simulink model "four_feet_simple_cdh"  (R2022b)
settings: Solver=FixedStepAuto  StartTime=0.0  StopTime=4  FixedStep=1e-4  MaxStep=1e-4  MinStep=1e-4  RelTol=1e-3  AbsTol=1e-3  EnableMultiTasking=on
undefined symbols (not defined in the file or in its folder): X, Y, Z
libraries: sm_lib x18, nesl_utility x7
settings Model: Creator=Administrator  LastModifiedBy=LiAn
settings SolverCC: AutoScaleAbsTol=off  AlgebraicLoopSolver=TrustRegion  MaxZcPerStep=1
settings DataIOCC: LimitDataPoints=on  MaxDataPoints=10000
settings OptimizationCC: LifeSpan=inf
settings DebuggingCC: UnconnectedInputMsg=warning  UnconnectedOutputMsg=warning  UnconnectedLineMsg=warning  AllowSymbolicDim=off  SFUnexpectedBacktrackingDiag=warning  SFNoUnconditionalDefaultTransitionDiag=warning  SFExecutionAtInitializationDiag=none  SFMachineParentedDataDiag=warning  ArithmeticOperatorsInVariantConditions=warning
settings ModelReferenceCC: EnableRefExpFcnMdlSchedulingChecks=on
settings SFSimCC: SimUseLocalCustomCode=off  CustomCodeUndefinedFunction=UseInterfaceOnly
settings RTWCC: RTWUseLocalCustomCode=off  DLArmComputeVersion=19.05
settings CodeAppCC: StateflowObjectComments=on
settings GRTTargetCC: TargetLangStandard=C89/C90 (ANSI)
settings ConfigComp: CovMetricSettings=dw  CovSaveCumulativeToWorkspaceVar=on  CovSaveSingleToWorkspaceVar=on  CovExternalEMLEnable=off  CovSFcnEnable=off
settings SimscapeCC: SimscapeLogType=all  SimscapeLogSimulationStatistics=on  SimscapeLogDataHistory=10000
settings DiagnosticsConfigSet: SimMechanicsRigidlyBoundBlock=warning

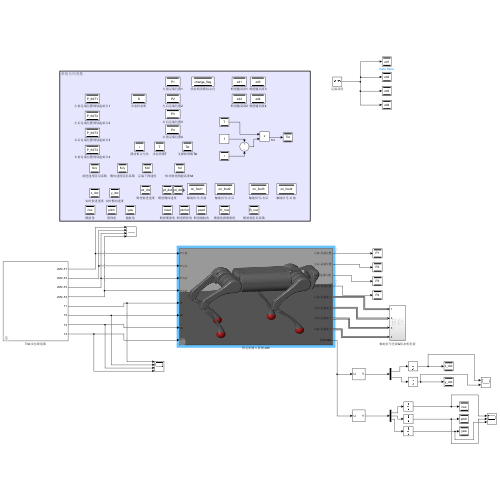
[thumbnail: Simulink's stored preview of the top-level diagram]
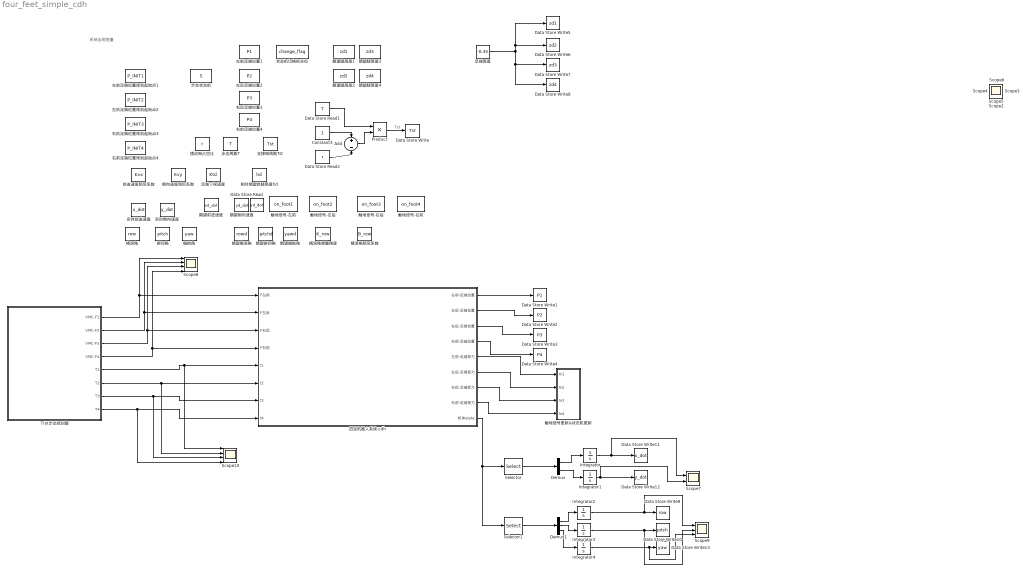
== system four_feet_simple_cdh ==
  note: 系统全局变量
  Add : Sum  Inputs=+-
  Constant3 : Constant
  Data Store Read : DataStoreRead  DataStoreName=yd_dot  IndexOptions=Index vector (dialog)  Indices=1  OutputSizes=1
  Data Store Read1 : DataStoreRead  DataStoreName=T  IndexOptions=Index vector (dialog)  Indices=1  OutputSizes=1
  Data Store Read2 : DataStoreRead  DataStoreName=r  IndexOptions=Index vector (dialog)  Indices=1  OutputSizes=1
  Data Store Write : DataStoreWrite  DataStoreName=Tst  IndexOptions=Index vector (dialog)  Indices=1  OutputSizes=1
  Data Store Write1 : DataStoreWrite  DataStoreName=P1  IndexOptions=Index vector (dialog)  Indices=1  OutputSizes=1
  Data Store Write10 : DataStoreWrite  DataStoreName=pitch  IndexOptions=Index vector (dialog)  Indices=1  OutputSizes=1
  Data Store Write11 : DataStoreWrite  DataStoreName=x_dot  IndexOptions=Index vector (dialog)  Indices=1  OutputSizes=1
  Data Store Write12 : DataStoreWrite  DataStoreName=y_dot  IndexOptions=Index vector (dialog)  Indices=1  OutputSizes=1
  Data Store Write13 : DataStoreWrite  DataStoreName=yaw  IndexOptions=Index vector (dialog)  Indices=1  OutputSizes=1
  Data Store Write2 : DataStoreWrite  DataStoreName=P2  IndexOptions=Index vector (dialog)  Indices=1  OutputSizes=1
  Data Store Write3 : DataStoreWrite  DataStoreName=P3  IndexOptions=Index vector (dialog)  Indices=1  OutputSizes=1
  Data Store Write4 : DataStoreWrite  DataStoreName=P4  IndexOptions=Index vector (dialog)  Indices=1  OutputSizes=1
  Data Store Write5 : DataStoreWrite  DataStoreName=zd1  IndexOptions=Index vector (dialog)  Indices=1  OutputSizes=1
  Data Store Write6 : DataStoreWrite  DataStoreName=zd2  IndexOptions=Index vector (dialog)  Indices=1  OutputSizes=1
  Data Store Write7 : DataStoreWrite  DataStoreName=zd3  IndexOptions=Index vector (dialog)  Indices=1  OutputSizes=1
  Data Store Write8 : DataStoreWrite  DataStoreName=zd4  IndexOptions=Index vector (dialog)  Indices=1  OutputSizes=1
  Data Store Write9 : DataStoreWrite  DataStoreName=row  IndexOptions=Index vector (dialog)  Indices=1  OutputSizes=1
  Demux : Demux  Outputs=2
  Demux1 : Demux  Outputs=3
  Integrator{,1..4} (5 alike) : Integrator
  Product : Product
  Scope10 : Scope  NumInputPorts=4
  Scope7 : Scope  NumInputPorts=2
  Scope8 : Scope  NumInputPorts=4
  Scope9 : Scope  NumInputPorts=3
  Selector : Selector  InputPortWidth=6  IndexOptions=Index vector (dialog)  Indices=[1 2]  OutputSizes=1
  Selector1 : Selector  InputPortWidth=6  IndexOptions=Index vector (dialog)  Indices=[4 5 6]  OutputSizes=1
  Trot步态规划器 : Subsystem  mask{P=2000, D=5}
      mask prompts: P "比例系数P"; D "阻尼系数D"
      mask DialogControl ParameterGroupVar Prompt: 参数
  侧向速度阻尼系数 : DataStoreMemory  DataStoreName=Kvy  WriteAfterWriteMsg=warning  InitialValue=-0.05  ShowAdditionalParam=off
  俯仰角 : DataStoreMemory  DataStoreName=pitch  WriteAfterWriteMsg=warning  ShowAdditionalParam=off
  偏航角 : DataStoreMemory  DataStoreName=yaw  WriteAfterWriteMsg=warning  ShowAdditionalParam=off
  前进速度阻尼系数 : DataStoreMemory  DataStoreName=Kvx  WriteAfterWriteMsg=warning  InitialValue=-0.3  ShowAdditionalParam=off
  右前足端位置4 : DataStoreMemory  DataStoreName=P4  WriteAfterWriteMsg=warning  InitialValue=[0 -0.085 -0.3]  ShowAdditionalParam=off
  右前足端位置规划起始点4 : DataStoreMemory  DataStoreName=P_INIT4  WriteAfterWriteMsg=warning  InitialValue=[0 -0.085 -0.3]  ShowAdditionalParam=off
  右后足端位置3 : DataStoreMemory  DataStoreName=P3  WriteAfterWriteMsg=warning  InitialValue=[0 -0.085 -0.3]  ShowAdditionalParam=off
  右后足端位置规划起始点3 : DataStoreMemory  DataStoreName=P_INIT3  WriteAfterWriteMsg=warning  InitialValue=[0 -0.085 -0.3]  ShowAdditionalParam=off
  四足机器人系统-cdh : Subsystem  mask{L=0.365, W=0.1, H=0.020, l1=0.085, l2=0.20, l3=0.20, floor_x=2, floor_y=2, floor_h=0.05, h_init=0.4, damping=10, stiff=10000, friction_v=0.3, friction_p=0.7, P=100, D=-0.1}
      mask prompts: L "机体长度"; W "机体宽度"; H "机体高度"; l1 "腿部连杆1长度"; l2 "腿部连杆2长度"; l3 "腿部连杆3长度"; floor_x "地面长"; floor_y "地面宽"; floor_h "地面高"; h_init "一开始离地高度"; damping "接触阻尼"; stiff "接触刚度"; friction_v "动摩擦系数"; friction_p "静摩擦系数"; P "VMC 弹性系数"; D "VMC 阻尼系数"
      mask DialogControl ParameterGroupVar Prompt: 参数
      mask Display: image('$imagefile'); % 使用工具条上的 "编辑图像" 进行更改。
  实时侧向速度 : DataStoreMemory  DataStoreName=y_dot  WriteAfterWriteMsg=warning  ShowAdditionalParam=off
  实时前进速度 : DataStoreMemory  DataStoreName=x_dot  WriteAfterWriteMsg=warning  ShowAdditionalParam=off
  左前足端位置1 : DataStoreMemory  DataStoreName=P1  WriteAfterWriteMsg=warning  InitialValue=[0 -0.085 -0.3]  ShowAdditionalParam=off
  左前足端位置规划起始点1 : DataStoreMemory  DataStoreName=P_INIT1  WriteAfterWriteMsg=warning  InitialValue=[0 0.085 -0.3]  ShowAdditionalParam=off
  左后足端位置2 : DataStoreMemory  DataStoreName=P2  WriteAfterWriteMsg=warning  InitialValue=[0 -0.085 -0.3]  ShowAdditionalParam=off
  左后足端位置规划起始点2 : DataStoreMemory  DataStoreName=P_INIT2  WriteAfterWriteMsg=warning  InitialValue=[0 0.085 -0.3]  ShowAdditionalParam=off
  摆动相占空比 : DataStoreMemory  DataStoreName=r  WriteAfterWriteMsg=warning  InitialValue=0.5  ShowAdditionalParam=off
  支撑相周期Tst : DataStoreMemory  DataStoreName=Tst  WriteAfterWriteMsg=warning  InitialValue=2  ShowAdditionalParam=off
  期望侧向速度 : DataStoreMemory  DataStoreName=yd_dot  WriteAfterWriteMsg=warning  ShowAdditionalParam=off
  期望俯仰角 : DataStoreMemory  DataStoreName=pitchd  WriteAfterWriteMsg=warning  ShowAdditionalParam=off
  期望偏航角 : DataStoreMemory  DataStoreName=yawd  WriteAfterWriteMsg=warning  ShowAdditionalParam=off
  期望前进速度 : DataStoreMemory  DataStoreName=xd_dot  WriteAfterWriteMsg=warning  InitialValue=0.05  ShowAdditionalParam=off
  期望横滚角 : DataStoreMemory  DataStoreName=rowd  WriteAfterWriteMsg=warning  InitialValue=0.5  ShowAdditionalParam=off
  期望腿高度1 : DataStoreMemory  DataStoreName=zd1  WriteAfterWriteMsg=warning  InitialValue=-0.35  ShowAdditionalParam=off
  期望腿高度2 : DataStoreMemory  DataStoreName=zd2  WriteAfterWriteMsg=warning  InitialValue=-0.35  ShowAdditionalParam=off
  期望腿高度3 : DataStoreMemory  DataStoreName=zd3  WriteAfterWriteMsg=warning  InitialValue=-0.35  ShowAdditionalParam=off
  期望腿高度4 : DataStoreMemory  DataStoreName=zd4  WriteAfterWriteMsg=warning  InitialValue=-0.35  ShowAdditionalParam=off
  横滚角 : DataStoreMemory  DataStoreName=row  WriteAfterWriteMsg=warning  ShowAdditionalParam=off
  横滚角弹簧刚度 : DataStoreMemory  DataStoreName=K_row  WriteAfterWriteMsg=warning  ShowAdditionalParam=off
  横滚角阻尼系数 : DataStoreMemory  DataStoreName=B_row  WriteAfterWriteMsg=warning  ShowAdditionalParam=off
  步态周期T : DataStoreMemory  DataStoreName=T  WriteAfterWriteMsg=warning  InitialValue=0.5  ShowAdditionalParam=off
  步态状态机 : DataStoreMemory  DataStoreName=S  WriteAfterWriteMsg=warning  InitialValue=-1  ShowAdditionalParam=off
  状态机切换标志位 : DataStoreMemory  DataStoreName=change_flag  WriteAfterWriteMsg=warning  ShowAdditionalParam=off
  "相对期望抬腿高度hd " : DataStoreMemory  DataStoreName=hd  WriteAfterWriteMsg=warning  InitialValue=0.05  ShowAdditionalParam=off
  "触地信号-右前 " : DataStoreMemory  DataStoreName=on_foot4  WriteAfterWriteMsg=warning  ShowAdditionalParam=off
  触地信号-右后 : DataStoreMemory  DataStoreName=on_foot3  WriteAfterWriteMsg=warning  ShowAdditionalParam=off
  触地信号-左前 : DataStoreMemory  DataStoreName=on_foot1  WriteAfterWriteMsg=warning  ShowAdditionalParam=off
  触地信号-左后 : DataStoreMemory  DataStoreName=on_foot2  WriteAfterWriteMsg=warning  ShowAdditionalParam=off
  触地信号更新&状态机更新 : Subsystem
  足端下探速度 : DataStoreMemory  DataStoreName=Ktd  WriteAfterWriteMsg=warning  InitialValue=0.3  ShowAdditionalParam=off
  足端高度 : Constant  Value=-0.35
  Scope{,1..6} (7 alike) : Scope
  wires:
  Data Store Read1/1 -> Product/1
  Constant3/1 -> Add/1
  Add/1 -> Product/2
  Product/1 -> Data Store Write/1  "Tst"
  Data Store Read2/1 -> Add/2
  四足机器人系统-cdh/5(左前-足端受力) -> 触地信号更新&状态机更新/1(In1)
  四足机器人系统-cdh/6(左后-足端受力) -> 触地信号更新&状态机更新/2(In2)
  四足机器人系统-cdh/7(右后-足端受力) -> 触地信号更新&状态机更新/3(In3)
  四足机器人系统-cdh/8(右前-足端受力) -> 触地信号更新&状态机更新/4(In4)
  四足机器人系统-cdh/1(左前-足端位置) -> Data Store Write1/1
  四足机器人系统-cdh/2(左后-足端位置) -> Data Store Write2/1
  四足机器人系统-cdh/3("右后-足端位置 ") -> Data Store Write3/1
  四足机器人系统-cdh/4(右前-足端位置) -> Data Store Write4/1
  四足机器人系统-cdh/9(机体state) -> Selector1/1, Selector/1
  Selector/1 -> Demux/1
  Demux/1 -> Integrator/1
  Demux/2 -> Integrator1/1
  Integrator/1 -> Scope7/1, Data Store Write11/1
  Integrator1/1 -> Scope7/2, Data Store Write12/1
  Trot步态规划器/1(VMC-F1) -> 四足机器人系统-cdh/1(F左前), Scope8/1
  Trot步态规划器/2(VMC-F2) -> 四足机器人系统-cdh/2(F左后), Scope8/2
  Trot步态规划器/3(VMC-F3) -> 四足机器人系统-cdh/3("F右后 "), Scope8/3
  Trot步态规划器/4(VMC-F4) -> 四足机器人系统-cdh/4(F右前), Scope8/4
  足端高度/1 -> Data Store Write8/1, Data Store Write7/1, Data Store Write6/1, Data Store Write5/1
  Selector1/1 -> Demux1/1
  Demux1/1 -> Integrator2/1
  Demux1/2 -> Integrator3/1
  Demux1/3 -> Integrator4/1
  Integrator2/1 -> Scope9/1, Data Store Write9/1
  Integrator3/1 -> Scope9/2, Data Store Write10/1
  Integrator4/1 -> Scope9/3, Data Store Write13/1
  Trot步态规划器/5(T1) -> Scope10/1, 四足机器人系统-cdh/5(t1)
  Trot步态规划器/6(T2) -> Scope10/2, 四足机器人系统-cdh/6(t2)
  Trot步态规划器/7(T3) -> Scope10/3, 四足机器人系统-cdh/7(t3)
  Trot步态规划器/8(T4) -> Scope10/4, 四足机器人系统-cdh/8(t4)

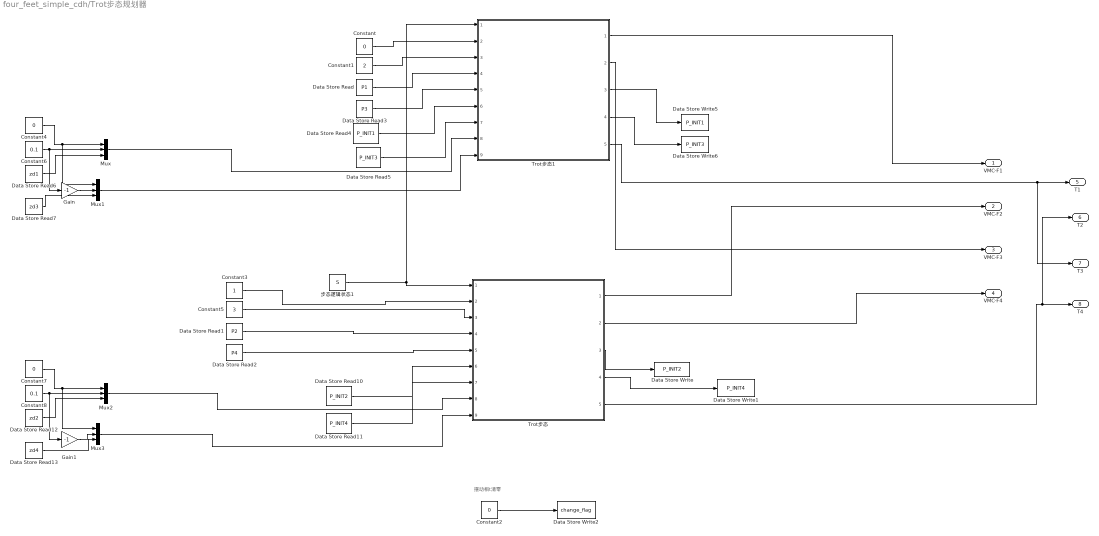
== system four_feet_simple_cdh/Trot步态规划器 ==
  note: 摆动相t清零
  Constant{,2,4,7} (4 alike) : Constant  Value=0
  Constant1 : Constant  Value=2
  Constant3 : Constant
  Constant5 : Constant  Value=3
  Constant6 : Constant  Value=0.1
  Constant8 : Constant  Value=0.1
  Data Store Read : DataStoreRead  DataStoreName=P1  IndexOptions=Index vector (dialog)  Indices=1  OutputSizes=1
  Data Store Read1 : DataStoreRead  DataStoreName=P2  IndexOptions=Index vector (dialog)  Indices=1  OutputSizes=1
  Data Store Read10 : DataStoreRead  DataStoreName=P_INIT2  IndexOptions=Index vector (dialog)  Indices=1  OutputSizes=1
  Data Store Read11 : DataStoreRead  DataStoreName=P_INIT4  IndexOptions=Index vector (dialog)  Indices=1  OutputSizes=1
  Data Store Read12 : DataStoreRead  DataStoreName=zd2  IndexOptions=Index vector (dialog)  Indices=1  OutputSizes=1
  Data Store Read13 : DataStoreRead  DataStoreName=zd4  IndexOptions=Index vector (dialog)  Indices=1  OutputSizes=1
  Data Store Read2 : DataStoreRead  DataStoreName=P4  IndexOptions=Index vector (dialog)  Indices=1  OutputSizes=1
  Data Store Read3 : DataStoreRead  DataStoreName=P3  IndexOptions=Index vector (dialog)  Indices=1  OutputSizes=1
  Data Store Read4 : DataStoreRead  DataStoreName=P_INIT1  IndexOptions=Index vector (dialog)  Indices=1  OutputSizes=1
  Data Store Read5 : DataStoreRead  DataStoreName=P_INIT3  IndexOptions=Index vector (dialog)  Indices=1  OutputSizes=1
  Data Store Read6 : DataStoreRead  DataStoreName=zd1  IndexOptions=Index vector (dialog)  Indices=1  OutputSizes=1
  Data Store Read7 : DataStoreRead  DataStoreName=zd3  IndexOptions=Index vector (dialog)  Indices=1  OutputSizes=1
  Data Store Write : DataStoreWrite  DataStoreName=P_INIT2  IndexOptions=Index vector (dialog)  Indices=1  OutputSizes=1
  Data Store Write1 : DataStoreWrite  DataStoreName=P_INIT4  IndexOptions=Index vector (dialog)  Indices=1  OutputSizes=1
  Data Store Write2 : DataStoreWrite  DataStoreName=change_flag  IndexOptions=Index vector (dialog)  Indices=1  OutputSizes=1
  Data Store Write5 : DataStoreWrite  DataStoreName=P_INIT1  IndexOptions=Index vector (dialog)  Indices=1  OutputSizes=1
  Data Store Write6 : DataStoreWrite  DataStoreName=P_INIT3  IndexOptions=Index vector (dialog)  Indices=1  OutputSizes=1
  Gain : Gain  Gain=-1
  Gain1 : Gain  Gain=-1
  Mux{,1..3} (4 alike) : Mux  Inputs=3
  Trot步态 : Subsystem  ReferencedSubsystem=Trot_planning
  Trot步态1 : Subsystem  ReferencedSubsystem=Trot_planning
  步态逻辑状态1 : DataStoreRead  DataStoreName=S  IndexOptions=Index vector (dialog)  Indices=1  OutputSizes=1
  VMC-F1 : Outport
  VMC-F2 : Outport  Port=2
  VMC-F3 : Outport  Port=3
  VMC-F4 : Outport  Port=4
  T1 : Outport  Port=5
  T2 : Outport  Port=6
  T3 : Outport  Port=7
  T4 : Outport  Port=8
  wires:
  Trot步态1/4 -> Data Store Write6/1
  Trot步态1/3 -> Data Store Write5/1
  步态逻辑状态1/1 -> Trot步态1/1, Trot步态/1
  Constant5/1 -> Trot步态/3
  Constant3/1 -> Trot步态/2
  Trot步态/3 -> Data Store Write/1
  Trot步态/4 -> Data Store Write1/1
  Trot步态/1 -> VMC-F2/1
  Trot步态/2 -> VMC-F4/1
  Constant/1 -> Trot步态1/2
  Constant1/1 -> Trot步态1/3
  Data Store Read/1 -> Trot步态1/4
  Data Store Read3/1 -> Trot步态1/5
  Data Store Read4/1 -> Trot步态1/6
  Data Store Read5/1 -> Trot步态1/7
  Trot步态1/1 -> VMC-F1/1
  Trot步态1/2 -> VMC-F3/1
  Constant2/1 -> Data Store Write2/1
  Data Store Read13/1 -> Mux3/3
  Gain1/1 -> Mux3/2
  Data Store Read12/1 -> Mux2/3
  Constant8/1 -> Gain1/1, Mux2/2
  Constant7/1 -> Mux2/1, Mux3/1
  Data Store Read7/1 -> Mux1/3
  Gain/1 -> Mux1/2
  Constant6/1 -> Mux/2, Gain/1
  Data Store Read6/1 -> Mux/3
  Constant4/1 -> Mux1/1, Mux/1
  Data Store Read10/1 -> Trot步态/6
  Data Store Read11/1 -> Trot步态/7
  Data Store Read1/1 -> Trot步态/4
  Data Store Read2/1 -> Trot步态/5
  Mux/1 -> Trot步态1/8
  Mux1/1 -> Trot步态1/9
  Mux2/1 -> Trot步态/8
  Mux3/1 -> Trot步态/9
  Trot步态1/5 -> T3/1, T1/1
  Trot步态/5 -> T2/1, T4/1

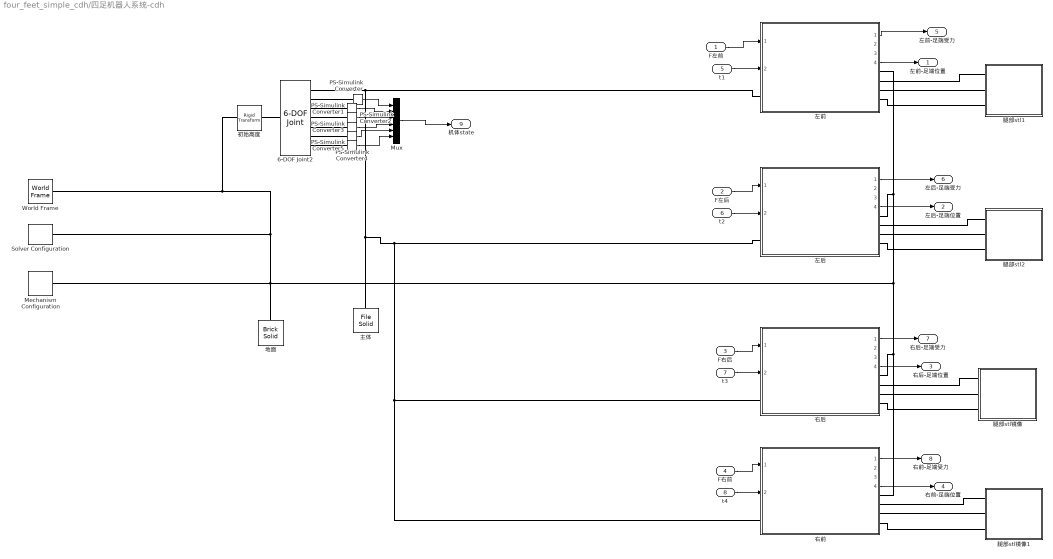
== system four_feet_simple_cdh/四足机器人系统-cdh ==
  F左前 : Inport
  F左后 : Inport  Port=2
  "F右后 " : Inport  Port=3
  F右前 : Inport  Port=4
  t1 : Inport  Port=5
  t2 : Inport  Port=6
  t3 : Inport  Port=7
  t4 : Inport  Port=8
  6-DOF Joint2 : sm_lib/Joints/6-DOF Joint  JointMode=Normal  SenseConstraintForce=off  SenseConstraintForceX=off  SenseConstraintForceY=off  SenseConstraintForceZ=off  SenseConstraintTorque=off  SenseConstraintTorqueX=off  SenseConstraintTorqueY=off  SenseConstraintTorqueZ=off  SenseTotalForce=off  SenseTotalForceX=off  SenseTotalForceY=off  SenseTotalForceZ=off  SenseTotalTorque=off  SenseTotalTorqueX=off  SenseTotalTorqueY=off  SenseTotalTorqueZ=off  CompositeWrenchDir=FollowerOnBase  CompositeWrenchFrame=BaseFrame  PxEquilibriumPosition=0  PxEquilibriumPositionUnits=m  PxSpringStiffness=0  PxSpringStiffnessUnits=N/m  PxDampingCoefficient=0  PxDampingCoefficientUnits=N/(m/s)  PxTorqueActuationMode=NoTorque  PxMotionActuationMode=ComputedMotion  PxSensePosition=off  PxSenseVelocity=off  PxSenseAcceleration=on  PxSenseTorqueForce=off  PxSenseLowerLimitTorqueForce=off  PxSenseUpperLimitTorqueForce=off  PxLowerLimitSpecify=off  PxLowerLimitBound=-1  PxLowerLimitBoundUnits=m  PxLowerLimitStiffness=1e6  PxLowerLimitStiffnessUnits=N/m  PxLowerLimitDamping=1e3  PxLowerLimitDampingUnits=N/(m/s)  PxLowerLimitTransitionRegionWidth=1e-4  PxLowerLimitTransitionRegionWidthUnits=m  PxUpperLimitSpecify=off  PxUpperLimitBound=1  PxUpperLimitBoundUnits=m  PxUpperLimitStiffness=1e6  PxUpperLimitStiffnessUnits=N/m  PxUpperLimitDamping=1e3  PxUpperLimitDampingUnits=N/(m/s)  PxUpperLimitTransitionRegionWidth=1e-4  PxUpperLimitTransitionRegionWidthUnits=m  PxPositionTargetSpecify=off  PxPositionTargetPriority=High  PxPositionTargetValue=0  PxPositionTargetValueUnits=m  PxVelocityTargetSpecify=off  PxVelocityTargetPriority=High  PxVelocityTargetValue=0  PxVelocityTargetValueUnits=m/s  PyEquilibriumPosition=0  PyEquilibriumPositionUnits=m  PySpringStiffness=0  PySpringStiffnessUnits=N/m  PyDampingCoefficient=0  PyDampingCoefficientUnits=N/(m/s)  PyTorqueActuationMode=NoTorque  PyMotionActuationMode=ComputedMotion  PySensePosition=off  PySenseVelocity=off  PySenseAcceleration=on  PySenseTorqueForce=off  PySenseLowerLimitTorqueForce=off  PySenseUpperLimitTorqueForce=off  PyLowerLimitSpecify=off  PyLowerLimitBound=-1  PyLowerLimitBoundUnits=m  PyLowerLimitStiffness=1e6  PyLowerLimitStiffnessUnits=N/m  PyLowerLimitDamping=1e3  PyLowerLimitDampingUnits=N/(m/s)  PyLowerLimitTransitionRegionWidth=1e-4  PyLowerLimitTransitionRegionWidthUnits=m  PyUpperLimitSpecify=off  PyUpperLimitBound=1  PyUpperLimitBoundUnits=m  PyUpperLimitStiffness=1e6  PyUpperLimitStiffnessUnits=N/m  PyUpperLimitDamping=1e3  PyUpperLimitDampingUnits=N/(m/s)  PyUpperLimitTransitionRegionWidth=1e-4  PyUpperLimitTransitionRegionWidthUnits=m  PyPositionTargetSpecify=off  PyPositionTargetPriority=High  PyPositionTargetValue=0  PyPositionTargetValueUnits=m  PyVelocityTargetSpecify=off  PyVelocityTargetPriority=High  PyVelocityTargetValue=0  PyVelocityTargetValueUnits=m/s  PzEquilibriumPosition=0  PzEquilibriumPositionUnits=m  PzSpringStiffness=0  PzSpringStiffnessUnits=N/m  PzDampingCoefficient=0  PzDampingCoefficientUnits=N/(m/s)  PzTorqueActuationMode=NoTorque  PzMotionActuationMode=ComputedMotion  PzSensePosition=off  PzSenseVelocity=off  PzSenseAcceleration=on  PzSenseTorqueForce=off  PzSenseLowerLimitTorqueForce=off  PzSenseUpperLimitTorqueForce=off  PzLowerLimitSpecify=off  PzLowerLimitBound=-1  PzLowerLimitBoundUnits=m  PzLowerLimitStiffness=1e6  PzLowerLimitStiffnessUnits=N/m  PzLowerLimitDamping=1e3  PzLowerLimitDampingUnits=N/(m/s)  PzLowerLimitTransitionRegionWidth=1e-4  PzLowerLimitTransitionRegionWidthUnits=m  PzUpperLimitSpecify=off  PzUpperLimitBound=1  PzUpperLimitBoundUnits=m  PzUpperLimitStiffness=1e6  PzUpperLimitStiffnessUnits=N/m  PzUpperLimitDamping=1e3  PzUpperLimitDampingUnits=N/(m/s)  PzUpperLimitTransitionRegionWidth=1e-4  PzUpperLimitTransitionRegionWidthUnits=m  PzPositionTargetSpecify=off  PzPositionTargetPriority=High  PzPositionTargetValue=0  PzPositionTargetValueUnits=m  PzVelocityTargetSpecify=off  PzVelocityTargetPriority=High  PzVelocityTargetValue=0  PzVelocityTargetValueUnits=m/s  SphEqPosRotationMethod=None  SphEqPosRotationAngleUnits=deg  SphEqPosRotationStandardAxis=+Z  SphEqPosRotationAngle=0.0  SphEqPosRotationArbitraryAxis=[0 0 1]  SphEqPosFollAlignAxisA=+X  SphEqPosBaseAlignAxisA=+Y  SphEqPosFollAlignAxisB=+Y  SphEqPosBaseAlignAxisB=+Z  SphEqPosRotationSequenceAxes=FollowerAxes  SphEqPosRotationSequence=XYX  SphEqPosRotationSequenceAngles=[0 0 0]  SphEqPosRotationSequenceAnglesUnits=deg  SphEqPosRotationMatrix=[1 0 0; 0 1 0; 0 0 1]  SphEqPosQuaternion=[1 0 0 0]  SphSpringStiffness=0  SphSpringStiffnessUnits=N*m/deg  SphDampingCoefficient=0  SphDampingCoefficientUnits=N*m/(deg/s)  SphActuateTorqueX=off  SphActuateTorqueY=off  SphActuateTorqueZ=off  SphActuateTorque=off  SphTorqueActuationMode=NoTorque  SphMotionActuationMode=ComputedMotion  SphActuationFrame=BaseFrame  SphSensePosition=off  SphSenseVelocityX=on  SphSenseVelocityY=on  SphSenseVelocityZ=on  SphSenseVelocity=off  SphSenseAccelerationX=off  SphSenseAccelerationY=off  SphSenseAccelerationZ=off  SphSenseAcceleration=off  SphSenseTorqueX=off  SphSenseTorqueY=off  SphSenseTorqueZ=off  SphSenseTorqueForce=off  SphSenseLowerLimitTorqueMag=off  SphSenseUpperLimitTorqueMag=off  SphSensingFrame=BaseFrame  SphLowerLimitSpecify=off  SphLowerLimitBound=15  SphLowerLimitBoundUnits=deg  SphLowerLimitStiffness=1e4  SphLowerLimitStiffnessUnits=N*m/deg  SphLowerLimitDamping=10  SphLowerLimitDampingUnits=N*m/(deg/s)  SphLowerLimitTransitionRegionWidth=0.1  SphLowerLimitTransitionRegionWidthUnits=deg  SphUpperLimitSpecify=off  SphUpperLimitBound=45  SphUpperLimitBoundUnits=deg  SphUpperLimitStiffness=1e4  SphUpperLimitStiffnessUnits=N*m/deg  SphUpperLimitDamping=10  SphUpperLimitDampingUnits=N*m/(deg/s)  SphUpperLimitTransitionRegionWidth=0.1  SphUpperLimitTransitionRegionWidthUnits=deg  SphPositionTargetRotationMethod=None  SphPositionTargetRotationAngleUnits=deg  SphPositionTargetRotationStandardAxis=+Z  SphPositionTargetRotationAngle=0.0  SphPositionTargetRotationArbitraryAxis=[0 0 1]  SphPositionTargetFollAlignAxisA=+X  SphPositionTargetBaseAlignAxisA=+Y  SphPositionTargetFollAlignAxisB=+Y  SphPositionTargetBaseAlignAxisB=+Z  SphPositionTargetRotationSequenceAxes=FollowerAxes  SphPositionTargetRotationSequence=XYX  SphPositionTargetRotationSequenceAngles=[0 0 0]  SphPositionTargetRotationSequenceAnglesUnits=deg  SphPositionTargetRotationMatrix=[1 0 0; 0 1 0; 0 0 1]  SphPositionTargetQuaternion=[1 0 0 0]  SphPositionTargetSpecify=off  SphPositionTargetPriority=High  SphVelocityTargetValue=[0 0 0]  SphVelocityTargetValueUnits=deg/s  SphVelocityTargetSpecify=off  SphVelocityTargetPriority=High  SphVelocityTargetInFollowerFrame=on
  Mechanism Configuration : sm_lib/Utilities/Mechanism Configuration  UniformGravity=Constant  GravityVector=[0 0 -9.80665]  GravityUnits=m/s^2  LinearizationDelta=0.001  JointModeTransitionNonlinearIterations=2
  Mux : Mux  Inputs=6
  PS-Simulink Converter{,1..5} (6 alike) : nesl_utility/PS-Simulink Converter  PhysicalDomain=network_engine_domain  SubClassName=ps_output  LeftPortType=input  RightPortType=output  PseudoPeriodic=off  Frequencies=[]  VectorFormat=inherit  Unit=inherit  AffineConversion=off
  Solver Configuration : nesl_utility/Solver Configuration  PhysicalDomain=network_engine_domain  SubClassName=solver  LeftPortType=input  RightPortType=generic  Tones=[]  Harmonics=[]  SimulateNoise=off  Profile=off  UseLocalSampling=off  EnableSwitchedLinearOptims=on  FrequencyDomain=off  UseCCode=off  RelTol=0.001  AbsTol=1e-06  MinStep=1e-09  ToWorkspace=off  RevertToSquareIcSolve=off  NumHomotopyIterations=100  PhasorMode=off  PhasorModeNumHarmonics=1  ConsistencySolver=NEWTON_XTOL_AFTER_FTOL  IndexReductionMethod=DerivativeReplacement  DoDC=off  ResidualTolerance=1e-09  ConsistencyTolSource=GLOBAL  ConsistencyAbsTol=0.001  ConsistencyRelTol=0.001  ConsistencyTolFactor=0.001  UseLocalSolver=off  LocalSolverChoice=NE_BACKWARD_EULER_ADVANCER  ResolveIndetEquations=on  FunctionEvalNumThread=1  LocalSolverSampleTime=0.001  DoFixedCost=off  MaxNonlinIter=3  MaxModeIter=2  ComputeImpulses=off  ImpulseIterations=2  LinearAlgebra=Sparse  LinearAlgebraNumThread=0  EquationFormulation=NE_TIME_EF  DelaysMemoryBudget=1024  AutomaticFiltering=on  FilteringTimeConstant=0.001  PartitionStorageMethod=AS_NEEDED  PartitionMemoryBudget=1024  PartitionMethod=FAST
  World Frame : sm_lib/Frames and Transforms/World Frame
  主体 : sm_lib/Body Elements/File Solid  ExtGeomFileName=unitree_stl\unitree_cad-main\unitree_cad-main\a1\trunk.STL  UnitType=Custom  ExtGeomFileUnits=m  StepReaderType=HEX  ExportConvexHullGeometry=off  InertiaType=CalculateFromGeometry  Mass=1  MassUnits=kg  CenterOfMass=[0 0 0]  CenterOfMassUnits=m  MomentsOfInertia=[1 1 1]  MomentsOfInertiaUnits=kg*m^2  ProductsOfInertia=[0 0 0]  ProductsOfInertiaUnits=kg*m^2  BasedOnType=Density  Density=1000  DensityUnits=kg/m^3  DoExposeReferenceFrame=on  SerializedFrames=<Frames/>  GraphicType=FromGeometry  MarkerShape=Sphere  MarkerSize=10  GraphicVisPropType=SimpleVisualProperties  GraphicDiffuseColor=[0.5 0.5 0.5]  GraphicSpecularColor=[0.5 0.5 0.5 1.0]  GraphicAmbientColor=[0.15 0.15 0.15 1.0]  GraphicEmissiveColor=[0.0 0.0 0.0 1.0]  GraphicShininess=75  GraphicOpacity=1.0
  初始高度 : sm_lib/Frames and Transforms/Rigid Transform  TranslationMethod=Cartesian  TranslationStandardOffset=0  TranslationLengthUnit=m  TranslationStandardAxis=+Z  TranslationCartesianOffset=[0 0 h_init]  TranslationROffset=0  TranslationROffsetUnits=m  TranslationZOffset=0  TranslationZOffsetUnits=m  TranslationThetaOffset=0  TranslationThetaOffsetUnits=deg  RotationMethod=StandardAxis  RotationAngleUnits=deg  RotationStandardAxis=+Y  RotationAngle=0  RotationArbitraryAxis=[0 0 1]  FollAlignAxisA=+X  BaseAlignAxisA=+Y  FollAlignAxisB=+Y  BaseAlignAxisB=+Z  RotationSequenceAxes=FollowerAxes  RotationSequence=XYX  RotationSequenceAngles=[0 0 0]  RotationSequenceAnglesUnits=deg  RotationMatrix=[1 0 0; 0 1 0; 0 0 1]  Quaternion=[1 0 0 0]
  右前 : Subsystem  ReferencedSubsystem=vmc_single_foot  P=50  D=-0.02  dir=-1  dir2=1
  "右后 " : Subsystem  ReferencedSubsystem=vmc_single_foot  P=50  D=-0.02  dir=-1  dir2=-1
  地面 : sm_lib/Body Elements/Brick Solid  GraphicAmbientColor=[0.15 0.15 0.15 1.0]  BasedOnType=Density  BrickDimensions=[floor_x floor_y floor_h*2]  BrickDimensionUnits=m  CenterOfMass=[0 0 0]  CenterOfMassUnits=m  GraphicDiffuseColor=[0.5 0.5 0.5]  Density=1000  DensityUnits=kg/m^3  DoExposeReferenceFrame=on  GraphicEmissiveColor=[0.0 0.0 0.0 1.0]  ExportEntireGeometry=off  SerializedFrames=<Frames/>  MarkerShape=Sphere  MarkerSize=10  GraphicType=FromGeometry  InertiaType=CalculateFromGeometry  Mass=1  MassUnits=kg  MomentsOfInertia=[1 1 1]  MomentsOfInertiaUnits=kg*m^2  GraphicOpacity=1.0  ProductsOfInertia=[0 0 0]  ProductsOfInertiaUnits=kg*m^2  GraphicShininess=75  GraphicSpecularColor=[0.5 0.5 0.5 1.0]  GraphicVisPropType=SimpleVisualProperties
  左前 : Subsystem  ReferencedSubsystem=vmc_single_foot  P=50  D=-0.02  dir=1  dir2=1
  左后 : Subsystem  ReferencedSubsystem=vmc_single_foot  P=50  D=-0.02  dir=1  dir2=-1
  腿部stl1 : Subsystem
  腿部stl2 : Subsystem
  腿部stl镜像 : Subsystem
  腿部stl镜像1 : Subsystem
  左前-足端位置 : Outport
  左后-足端位置 : Outport  Port=2
  "右后-足端位置 " : Outport  Port=3
  右前-足端位置 : Outport  Port=4
  左前-足端受力 : Outport  Port=5
  左后-足端受力 : Outport  Port=6
  右后-足端受力 : Outport  Port=7
  右前-足端受力 : Outport  Port=8
  机体state : Outport  Port=9
  wires:
  右前/4 -> 右前-足端位置/1
  "右后 "/4 -> "右后-足端位置 "/1
  左后/4 -> 左后-足端位置/1
  左前/4 -> 左前-足端位置/1
  F左前/1 -> 左前/1
  F左后/1 -> 左后/1
  "F右后 "/1 -> "右后 "/1
  F右前/1 -> 右前/1
  左前/1 -> 左前-足端受力/1
  左后/1 -> 左后-足端受力/1
  右前/1 -> 右前-足端受力/1
  "右后 "/1 -> 右后-足端受力/1
  PS-Simulink Converter/1 -> Mux/1
  PS-Simulink Converter1/1 -> Mux/2
  PS-Simulink Converter2/1 -> Mux/3
  PS-Simulink Converter3/1 -> Mux/4
  Mux/1 -> 机体state/1
  PS-Simulink Converter4/1 -> Mux/5
  PS-Simulink Converter5/1 -> Mux/6
  t1/1 -> 左前/2
  t2/1 -> 左后/2
  t3/1 -> "右后 "/2
  t4/1 -> 右前/2
  connections:
  左前/RConn2 -- 腿部stl1/LConn1
  左前/RConn3 -- 腿部stl1/LConn2
  左前/RConn4 -- 腿部stl1/LConn3
  腿部stl2/LConn3 -- 左后/RConn4
  腿部stl2/LConn2 -- 左后/RConn3
  腿部stl2/LConn1 -- 左后/RConn2
  腿部stl镜像1/LConn1 -- 右前/RConn2
  腿部stl镜像1/LConn2 -- 右前/RConn3
  腿部stl镜像1/LConn3 -- 右前/RConn4
  腿部stl镜像/LConn1 -- "右后 "/RConn2
  腿部stl镜像/LConn2 -- "右后 "/RConn3
  腿部stl镜像/LConn3 -- "右后 "/RConn4
  初始高度/LConn1 -- World Frame/RConn1 -- Solver Configuration/RConn1 -- Mechanism Configuration/RConn1 -- 地面/RConn1 -- 右前/RConn1 -- "右后 "/RConn1 -- 左前/RConn1 -- 左后/RConn1
  "右后 "/LConn1 -- 6-DOF Joint2/RConn1 -- 左前/LConn1 -- 主体/RConn1 -- 左后/LConn1 -- 右前/LConn1
  初始高度/RConn1 -- 6-DOF Joint2/LConn1
  PS-Simulink Converter/LConn1 -- 6-DOF Joint2/RConn2
  PS-Simulink Converter1/LConn1 -- 6-DOF Joint2/RConn3
  PS-Simulink Converter2/LConn1 -- 6-DOF Joint2/RConn4
  6-DOF Joint2/RConn5 -- PS-Simulink Converter3/LConn1
  6-DOF Joint2/RConn6 -- PS-Simulink Converter4/LConn1
  6-DOF Joint2/RConn7 -- PS-Simulink Converter5/LConn1

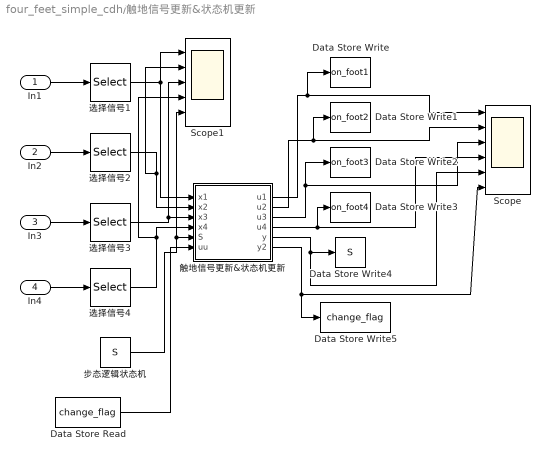
== system four_feet_simple_cdh/触地信号更新&状态机更新 ==
  In1 : Inport
  In2 : Inport  Port=2
  In3 : Inport  Port=3
  In4 : Inport  Port=4
  Data Store Read : DataStoreRead  DataStoreName=change_flag  IndexOptions=Index vector (dialog)  Indices=1  OutputSizes=1
  Data Store Write : DataStoreWrite  DataStoreName=on_foot1  IndexOptions=Index vector (dialog)  Indices=1  OutputSizes=1
  Data Store Write1 : DataStoreWrite  DataStoreName=on_foot2  IndexOptions=Index vector (dialog)  Indices=1  OutputSizes=1
  Data Store Write2 : DataStoreWrite  DataStoreName=on_foot3  IndexOptions=Index vector (dialog)  Indices=1  OutputSizes=1
  Data Store Write3 : DataStoreWrite  DataStoreName=on_foot4  IndexOptions=Index vector (dialog)  Indices=1  OutputSizes=1
  Data Store Write4 : DataStoreWrite  DataStoreName=S  IndexOptions=Index vector (dialog)  Indices=1  OutputSizes=1
  Data Store Write5 : DataStoreWrite  DataStoreName=change_flag  IndexOptions=Index vector (dialog)  Indices=1  OutputSizes=1
  Scope : Scope  NumInputPorts=6
  Scope1 : Scope  NumInputPorts=5
  步态逻辑状态机 : DataStoreRead  DataStoreName=S  IndexOptions=Index vector (dialog)  Indices=1  OutputSizes=1
  触地信号更新&状态机更新 : MATLAB Function  TreatAsAtomicUnit=on
  选择信号{1..4} (4 alike) : Selector  InputPortWidth=11  IndexOptions=Index vector (dialog)  Indices=1  OutputSizes=1
  wires:
  选择信号4/1 -> 触地信号更新&状态机更新/4(x4), Scope1/4
  In1/1 -> 选择信号1/1
  In3/1 -> 选择信号3/1
  In2/1 -> 选择信号2/1
  In4/1 -> 选择信号4/1
  选择信号1/1 -> Scope1/1, 触地信号更新&状态机更新/1(x1)
  选择信号3/1 -> Scope1/3, 触地信号更新&状态机更新/3(x3)
  选择信号2/1 -> Scope1/2, 触地信号更新&状态机更新/2(x2)
  步态逻辑状态机/1 -> Scope1/5, 触地信号更新&状态机更新/5(S)
  触地信号更新&状态机更新/1(u1) -> Data Store Write/1, Scope/1
  触地信号更新&状态机更新/2(u2) -> Data Store Write1/1, Scope/2
  触地信号更新&状态机更新/4(u4) -> Data Store Write3/1, Scope/4
  触地信号更新&状态机更新/5(y) -> Scope/5, Data Store Write4/1
  触地信号更新&状态机更新/3(u3) -> Data Store Write2/1, Scope/3
  触地信号更新&状态机更新/6(y2) -> Scope/6, Data Store Write5/1
  Data Store Read/1 -> 触地信号更新&状态机更新/6(uu)

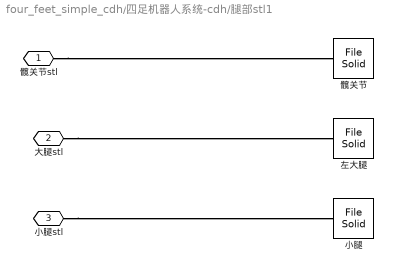
== system four_feet_simple_cdh/四足机器人系统-cdh/腿部stl1 ==
  小腿 : sm_lib/Body Elements/File Solid  ExtGeomFileName=unitree_stl\unitree_cad-main\unitree_cad-main\a1\calf.STL  UnitType=Custom  ExtGeomFileUnits=m  StepReaderType=HEX  ExportConvexHullGeometry=off  InertiaType=CalculateFromGeometry  Mass=1  MassUnits=kg  CenterOfMass=[0 0 0]  CenterOfMassUnits=m  MomentsOfInertia=[1 1 1]  MomentsOfInertiaUnits=kg*m^2  ProductsOfInertia=[0 0 0]  ProductsOfInertiaUnits=kg*m^2  BasedOnType=Density  Density=1000  DensityUnits=kg/m^3  DoExposeReferenceFrame=off  SerializedFrames=<Frames><Frame><Id>Frame1</Id><Value><Name>F1</Name><Origin><Source>ReferenceFrame</Source><FeatureName></FeatureName></Origin><PrimaryAxis><DefinedDirection>+Z</DefinedDirection><Source>ReferenceFrame</Source><SourceDirection>+Y</SourceDirection><FeatureName></FeatureName></PrimaryAxis><SecondaryAxis><DefinedDirection>+X</DefinedDirection><Source>ReferenceFrame</Source><SourceDirection>-Z</SourceDirection><FeatureName></FeatureName></SecondaryAxis></Value></Frame></Frames>  GraphicType=FromGeometry  MarkerShape=Sphere  MarkerSize=10  GraphicVisPropType=SimpleVisualProperties  GraphicDiffuseColor=[0.5 0.5 0.5]  GraphicSpecularColor=[0.5 0.5 0.5 1.0]  GraphicAmbientColor=[0.15 0.15 0.15 1.0]  GraphicEmissiveColor=[0.0 0.0 0.0 1.0]  GraphicShininess=75  GraphicOpacity=1.0
  左大腿 : sm_lib/Body Elements/File Solid  ExtGeomFileName=unitree_stl\unitree_cad-main\unitree_cad-main\a1\thigh_left.STL  UnitType=Custom  ExtGeomFileUnits=m  StepReaderType=HEX  ExportConvexHullGeometry=off  InertiaType=CalculateFromGeometry  Mass=1  MassUnits=kg  CenterOfMass=[0 0 0]  CenterOfMassUnits=m  MomentsOfInertia=[1 1 1]  MomentsOfInertiaUnits=kg*m^2  ProductsOfInertia=[0 0 0]  ProductsOfInertiaUnits=kg*m^2  BasedOnType=Density  Density=1000  DensityUnits=kg/m^3  DoExposeReferenceFrame=off  SerializedFrames=<Frames><Frame><Id>Frame1</Id><Value><Name>F1</Name><Origin><Source>ReferenceFrame</Source><FeatureName></FeatureName></Origin><PrimaryAxis><DefinedDirection>+Z</DefinedDirection><Source>ReferenceFrame</Source><SourceDirection>+Y</SourceDirection><FeatureName></FeatureName></PrimaryAxis><SecondaryAxis><DefinedDirection>+X</DefinedDirection><Source>ReferenceFrame</Source><SourceDirection>-Z</SourceDirection><FeatureName></FeatureName></SecondaryAxis></Value></Frame></Frames>  GraphicType=FromGeometry  MarkerShape=Sphere  MarkerSize=10  GraphicVisPropType=SimpleVisualProperties  GraphicDiffuseColor=[0.5 0.5 0.5]  GraphicSpecularColor=[0.5 0.5 0.5 1.0]  GraphicAmbientColor=[0.15 0.15 0.15 1.0]  GraphicEmissiveColor=[0.0 0.0 0.0 1.0]  GraphicShininess=75  GraphicOpacity=1.0
  髋关节 : sm_lib/Body Elements/File Solid  ExtGeomFileName=unitree_stl\unitree_cad-main\unitree_cad-main\a1\hip.STL  UnitType=Custom  ExtGeomFileUnits=m  StepReaderType=HEX  ExportConvexHullGeometry=off  InertiaType=CalculateFromGeometry  Mass=1  MassUnits=kg  CenterOfMass=[0 0 0]  CenterOfMassUnits=m  MomentsOfInertia=[1 1 1]  MomentsOfInertiaUnits=kg*m^2  ProductsOfInertia=[0 0 0]  ProductsOfInertiaUnits=kg*m^2  BasedOnType=Density  Density=1000  DensityUnits=kg/m^3  DoExposeReferenceFrame=off  SerializedFrames=<Frames><Frame><Id>Frame1</Id><Value><Name>F1</Name><Origin><Source>ReferenceFrame</Source><FeatureName></FeatureName></Origin><PrimaryAxis><DefinedDirection>+Z</DefinedDirection><Source>ReferenceFrame</Source><SourceDirection>+X</SourceDirection><FeatureName></FeatureName></PrimaryAxis><SecondaryAxis><DefinedDirection>+X</DefinedDirection><Source>ReferenceFrame</Source><SourceDirection>-Z</SourceDirection><FeatureName></FeatureName></SecondaryAxis></Value></Frame></Frames>  GraphicType=FromGeometry  MarkerShape=Sphere  MarkerSize=10  GraphicVisPropType=SimpleVisualProperties  GraphicDiffuseColor=[0.5 0.5 0.5]  GraphicSpecularColor=[0.5 0.5 0.5 1.0]  GraphicAmbientColor=[0.15 0.15 0.15 1.0]  GraphicEmissiveColor=[0.0 0.0 0.0 1.0]  GraphicShininess=75  GraphicOpacity=1.0
  "髋关节stl " : PMIOPort  Side=Left
  "大腿stl " : PMIOPort  Port=2  Side=Left
  "小腿stl " : PMIOPort  Port=3  Side=Left
  connections:
  "大腿stl "/RConn1 -- 左大腿/LConn1
  "髋关节stl "/RConn1 -- 髋关节/LConn1
  "小腿stl "/RConn1 -- 小腿/LConn1

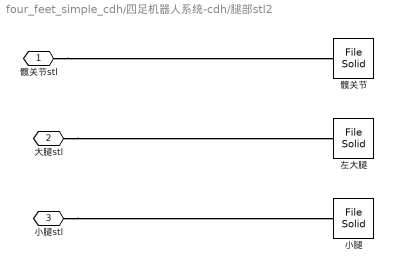
== system four_feet_simple_cdh/四足机器人系统-cdh/腿部stl2 ==
  小腿 : sm_lib/Body Elements/File Solid  ExtGeomFileName=unitree_stl\unitree_cad-main\unitree_cad-main\a1\calf.STL  UnitType=Custom  ExtGeomFileUnits=m  StepReaderType=HEX  ExportConvexHullGeometry=off  InertiaType=CalculateFromGeometry  Mass=1  MassUnits=kg  CenterOfMass=[0 0 0]  CenterOfMassUnits=m  MomentsOfInertia=[1 1 1]  MomentsOfInertiaUnits=kg*m^2  ProductsOfInertia=[0 0 0]  ProductsOfInertiaUnits=kg*m^2  BasedOnType=Density  Density=1000  DensityUnits=kg/m^3  DoExposeReferenceFrame=off  SerializedFrames=<Frames><Frame><Id>Frame1</Id><Value><Name>F1</Name><Origin><Source>ReferenceFrame</Source><FeatureName></FeatureName></Origin><PrimaryAxis><DefinedDirection>+Z</DefinedDirection><Source>ReferenceFrame</Source><SourceDirection>+Y</SourceDirection><FeatureName></FeatureName></PrimaryAxis><SecondaryAxis><DefinedDirection>+X</DefinedDirection><Source>ReferenceFrame</Source><SourceDirection>-Z</SourceDirection><FeatureName></FeatureName></SecondaryAxis></Value></Frame></Frames>  GraphicType=FromGeometry  MarkerShape=Sphere  MarkerSize=10  GraphicVisPropType=SimpleVisualProperties  GraphicDiffuseColor=[0.5 0.5 0.5]  GraphicSpecularColor=[0.5 0.5 0.5 1.0]  GraphicAmbientColor=[0.15 0.15 0.15 1.0]  GraphicEmissiveColor=[0.0 0.0 0.0 1.0]  GraphicShininess=75  GraphicOpacity=1.0
  左大腿 : sm_lib/Body Elements/File Solid  ExtGeomFileName=unitree_stl\unitree_cad-main\unitree_cad-main\a1\thigh_left.STL  UnitType=Custom  ExtGeomFileUnits=m  StepReaderType=HEX  ExportConvexHullGeometry=off  InertiaType=CalculateFromGeometry  Mass=1  MassUnits=kg  CenterOfMass=[0 0 0]  CenterOfMassUnits=m  MomentsOfInertia=[1 1 1]  MomentsOfInertiaUnits=kg*m^2  ProductsOfInertia=[0 0 0]  ProductsOfInertiaUnits=kg*m^2  BasedOnType=Density  Density=1000  DensityUnits=kg/m^3  DoExposeReferenceFrame=off  SerializedFrames=<Frames><Frame><Id>Frame1</Id><Value><Name>F1</Name><Origin><Source>ReferenceFrame</Source><FeatureName></FeatureName></Origin><PrimaryAxis><DefinedDirection>+Z</DefinedDirection><Source>ReferenceFrame</Source><SourceDirection>+Y</SourceDirection><FeatureName></FeatureName></PrimaryAxis><SecondaryAxis><DefinedDirection>+X</DefinedDirection><Source>ReferenceFrame</Source><SourceDirection>-Z</SourceDirection><FeatureName></FeatureName></SecondaryAxis></Value></Frame></Frames>  GraphicType=FromGeometry  MarkerShape=Sphere  MarkerSize=10  GraphicVisPropType=SimpleVisualProperties  GraphicDiffuseColor=[0.5 0.5 0.5]  GraphicSpecularColor=[0.5 0.5 0.5 1.0]  GraphicAmbientColor=[0.15 0.15 0.15 1.0]  GraphicEmissiveColor=[0.0 0.0 0.0 1.0]  GraphicShininess=75  GraphicOpacity=1.0
  髋关节 : sm_lib/Body Elements/File Solid  ExtGeomFileName=unitree_stl\unitree_cad-main\unitree_cad-main\a1\hip.STL  UnitType=Custom  ExtGeomFileUnits=m  StepReaderType=HEX  ExportConvexHullGeometry=off  InertiaType=CalculateFromGeometry  Mass=1  MassUnits=kg  CenterOfMass=[0 0 0]  CenterOfMassUnits=m  MomentsOfInertia=[1 1 1]  MomentsOfInertiaUnits=kg*m^2  ProductsOfInertia=[0 0 0]  ProductsOfInertiaUnits=kg*m^2  BasedOnType=Density  Density=1000  DensityUnits=kg/m^3  DoExposeReferenceFrame=off  SerializedFrames=<Frames><Frame><Id>Frame1</Id><Value><Name>F1</Name><Origin><Source>ReferenceFrame</Source><FeatureName></FeatureName></Origin><PrimaryAxis><DefinedDirection>+Z</DefinedDirection><Source>ReferenceFrame</Source><SourceDirection>-X</SourceDirection><FeatureName></FeatureName></PrimaryAxis><SecondaryAxis><DefinedDirection>+X</DefinedDirection><Source>ReferenceFrame</Source><SourceDirection>-Z</SourceDirection><FeatureName></FeatureName></SecondaryAxis></Value></Frame></Frames>  GraphicType=FromGeometry  MarkerShape=Sphere  MarkerSize=10  GraphicVisPropType=SimpleVisualProperties  GraphicDiffuseColor=[0.5 0.5 0.5]  GraphicSpecularColor=[0.5 0.5 0.5 1.0]  GraphicAmbientColor=[0.15 0.15 0.15 1.0]  GraphicEmissiveColor=[0.0 0.0 0.0 1.0]  GraphicShininess=75  GraphicOpacity=1.0
  "髋关节stl " : PMIOPort  Side=Left
  "大腿stl " : PMIOPort  Port=2  Side=Left
  "小腿stl " : PMIOPort  Port=3  Side=Left
  connections:
  "小腿stl "/RConn1 -- 小腿/LConn1
  "髋关节stl "/RConn1 -- 髋关节/LConn1
  "大腿stl "/RConn1 -- 左大腿/LConn1

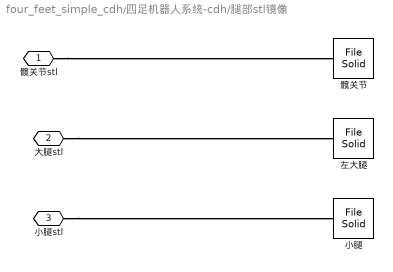
== system four_feet_simple_cdh/四足机器人系统-cdh/腿部stl镜像 ==
  小腿 : sm_lib/Body Elements/File Solid  ExtGeomFileName=unitree_stl\unitree_cad-main\unitree_cad-main\a1\calf.STL  UnitType=Custom  ExtGeomFileUnits=m  StepReaderType=HEX  ExportConvexHullGeometry=off  InertiaType=CalculateFromGeometry  Mass=1  MassUnits=kg  CenterOfMass=[0 0 0]  CenterOfMassUnits=m  MomentsOfInertia=[1 1 1]  MomentsOfInertiaUnits=kg*m^2  ProductsOfInertia=[0 0 0]  ProductsOfInertiaUnits=kg*m^2  BasedOnType=Density  Density=1000  DensityUnits=kg/m^3  DoExposeReferenceFrame=off  SerializedFrames=<Frames><Frame><Id>Frame1</Id><Value><Name>F1</Name><Origin><Source>ReferenceFrame</Source><FeatureName></FeatureName></Origin><PrimaryAxis><DefinedDirection>+Z</DefinedDirection><Source>ReferenceFrame</Source><SourceDirection>+Y</SourceDirection><FeatureName></FeatureName></PrimaryAxis><SecondaryAxis><DefinedDirection>+X</DefinedDirection><Source>ReferenceFrame</Source><SourceDirection>-Z</SourceDirection><FeatureName></FeatureName></SecondaryAxis></Value></Frame></Frames>  GraphicType=FromGeometry  MarkerShape=Sphere  MarkerSize=10  GraphicVisPropType=SimpleVisualProperties  GraphicDiffuseColor=[0.5 0.5 0.5]  GraphicSpecularColor=[0.5 0.5 0.5 1.0]  GraphicAmbientColor=[0.15 0.15 0.15 1.0]  GraphicEmissiveColor=[0.0 0.0 0.0 1.0]  GraphicShininess=75  GraphicOpacity=1.0
  左大腿 : sm_lib/Body Elements/File Solid  ExtGeomFileName=unitree_stl\unitree_cad-main\unitree_cad-main\a1\thigh_right.STL  UnitType=Custom  ExtGeomFileUnits=m  StepReaderType=HEX  ExportConvexHullGeometry=off  InertiaType=CalculateFromGeometry  Mass=1  MassUnits=kg  CenterOfMass=[0 0 0]  CenterOfMassUnits=m  MomentsOfInertia=[1 1 1]  MomentsOfInertiaUnits=kg*m^2  ProductsOfInertia=[0 0 0]  ProductsOfInertiaUnits=kg*m^2  BasedOnType=Density  Density=1000  DensityUnits=kg/m^3  DoExposeReferenceFrame=off  SerializedFrames=<Frames><Frame><Id>Frame1</Id><Value><Name>F1</Name><Origin><Source>ReferenceFrame</Source><FeatureName></FeatureName></Origin><PrimaryAxis><DefinedDirection>+Z</DefinedDirection><Source>ReferenceFrame</Source><SourceDirection>+Y</SourceDirection><FeatureName></FeatureName></PrimaryAxis><SecondaryAxis><DefinedDirection>+X</DefinedDirection><Source>ReferenceFrame</Source><SourceDirection>-Z</SourceDirection><FeatureName></FeatureName></SecondaryAxis></Value></Frame></Frames>  GraphicType=FromGeometry  MarkerShape=Sphere  MarkerSize=10  GraphicVisPropType=SimpleVisualProperties  GraphicDiffuseColor=[0.5 0.5 0.5]  GraphicSpecularColor=[0.5 0.5 0.5 1.0]  GraphicAmbientColor=[0.15 0.15 0.15 1.0]  GraphicEmissiveColor=[0.0 0.0 0.0 1.0]  GraphicShininess=75  GraphicOpacity=1.0
  髋关节 : sm_lib/Body Elements/File Solid  ExtGeomFileName=unitree_stl\unitree_cad-main\unitree_cad-main\a1\hip.STL  UnitType=Custom  ExtGeomFileUnits=m  StepReaderType=HEX  ExportConvexHullGeometry=off  InertiaType=CalculateFromGeometry  Mass=1  MassUnits=kg  CenterOfMass=[0 0 0]  CenterOfMassUnits=m  MomentsOfInertia=[1 1 1]  MomentsOfInertiaUnits=kg*m^2  ProductsOfInertia=[0 0 0]  ProductsOfInertiaUnits=kg*m^2  BasedOnType=Density  Density=1000  DensityUnits=kg/m^3  DoExposeReferenceFrame=off  SerializedFrames=<Frames><Frame><Id>Frame1</Id><Value><Name>F1</Name><Origin><Source>ReferenceFrame</Source><FeatureName></FeatureName></Origin><PrimaryAxis><DefinedDirection>+Z</DefinedDirection><Source>ReferenceFrame</Source><SourceDirection>-X</SourceDirection><FeatureName></FeatureName></PrimaryAxis><SecondaryAxis><DefinedDirection>+X</DefinedDirection><Source>ReferenceFrame</Source><SourceDirection>-Z</SourceDirection><FeatureName></FeatureName></SecondaryAxis></Value></Frame></Frames>  GraphicType=FromGeometry  MarkerShape=Sphere  MarkerSize=10  GraphicVisPropType=SimpleVisualProperties  GraphicDiffuseColor=[0.5 0.5 0.5]  GraphicSpecularColor=[0.5 0.5 0.5 1.0]  GraphicAmbientColor=[0.15 0.15 0.15 1.0]  GraphicEmissiveColor=[0.0 0.0 0.0 1.0]  GraphicShininess=75  GraphicOpacity=1.0
  "髋关节stl " : PMIOPort  Side=Left
  "大腿stl " : PMIOPort  Port=2  Side=Left
  "小腿stl " : PMIOPort  Port=3  Side=Left
  connections:
  "大腿stl "/RConn1 -- 左大腿/LConn1
  "髋关节stl "/RConn1 -- 髋关节/LConn1
  "小腿stl "/RConn1 -- 小腿/LConn1

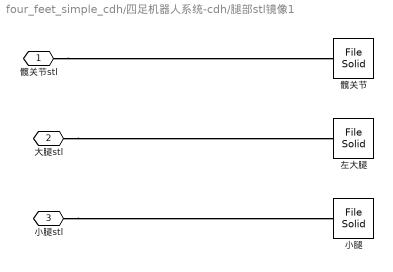
== system four_feet_simple_cdh/四足机器人系统-cdh/腿部stl镜像1 ==
  小腿 : sm_lib/Body Elements/File Solid  ExtGeomFileName=unitree_stl\unitree_cad-main\unitree_cad-main\a1\calf.STL  UnitType=Custom  ExtGeomFileUnits=m  StepReaderType=HEX  ExportConvexHullGeometry=off  InertiaType=CalculateFromGeometry  Mass=1  MassUnits=kg  CenterOfMass=[0 0 0]  CenterOfMassUnits=m  MomentsOfInertia=[1 1 1]  MomentsOfInertiaUnits=kg*m^2  ProductsOfInertia=[0 0 0]  ProductsOfInertiaUnits=kg*m^2  BasedOnType=Density  Density=1000  DensityUnits=kg/m^3  DoExposeReferenceFrame=off  SerializedFrames=<Frames><Frame><Id>Frame1</Id><Value><Name>F1</Name><Origin><Source>ReferenceFrame</Source><FeatureName></FeatureName></Origin><PrimaryAxis><DefinedDirection>+Z</DefinedDirection><Source>ReferenceFrame</Source><SourceDirection>+Y</SourceDirection><FeatureName></FeatureName></PrimaryAxis><SecondaryAxis><DefinedDirection>+X</DefinedDirection><Source>ReferenceFrame</Source><SourceDirection>-Z</SourceDirection><FeatureName></FeatureName></SecondaryAxis></Value></Frame></Frames>  GraphicType=FromGeometry  MarkerShape=Sphere  MarkerSize=10  GraphicVisPropType=SimpleVisualProperties  GraphicDiffuseColor=[0.5 0.5 0.5]  GraphicSpecularColor=[0.5 0.5 0.5 1.0]  GraphicAmbientColor=[0.15 0.15 0.15 1.0]  GraphicEmissiveColor=[0.0 0.0 0.0 1.0]  GraphicShininess=75  GraphicOpacity=1.0
  左大腿 : sm_lib/Body Elements/File Solid  ExtGeomFileName=unitree_stl\unitree_cad-main\unitree_cad-main\a1\thigh_right.STL  UnitType=Custom  ExtGeomFileUnits=m  StepReaderType=HEX  ExportConvexHullGeometry=off  InertiaType=CalculateFromGeometry  Mass=1  MassUnits=kg  CenterOfMass=[0 0 0]  CenterOfMassUnits=m  MomentsOfInertia=[1 1 1]  MomentsOfInertiaUnits=kg*m^2  ProductsOfInertia=[0 0 0]  ProductsOfInertiaUnits=kg*m^2  BasedOnType=Density  Density=1000  DensityUnits=kg/m^3  DoExposeReferenceFrame=off  SerializedFrames=<Frames><Frame><Id>Frame1</Id><Value><Name>F1</Name><Origin><Source>ReferenceFrame</Source><FeatureName></FeatureName></Origin><PrimaryAxis><DefinedDirection>+Z</DefinedDirection><Source>ReferenceFrame</Source><SourceDirection>+Y</SourceDirection><FeatureName></FeatureName></PrimaryAxis><SecondaryAxis><DefinedDirection>+X</DefinedDirection><Source>ReferenceFrame</Source><SourceDirection>-Z</SourceDirection><FeatureName></FeatureName></SecondaryAxis></Value></Frame></Frames>  GraphicType=FromGeometry  MarkerShape=Sphere  MarkerSize=10  GraphicVisPropType=SimpleVisualProperties  GraphicDiffuseColor=[0.5 0.5 0.5]  GraphicSpecularColor=[0.5 0.5 0.5 1.0]  GraphicAmbientColor=[0.15 0.15 0.15 1.0]  GraphicEmissiveColor=[0.0 0.0 0.0 1.0]  GraphicShininess=75  GraphicOpacity=1.0
  髋关节 : sm_lib/Body Elements/File Solid  ExtGeomFileName=unitree_stl\unitree_cad-main\unitree_cad-main\a1\hip.STL  UnitType=Custom  ExtGeomFileUnits=m  StepReaderType=HEX  ExportConvexHullGeometry=off  InertiaType=CalculateFromGeometry  Mass=1  MassUnits=kg  CenterOfMass=[0 0 0]  CenterOfMassUnits=m  MomentsOfInertia=[1 1 1]  MomentsOfInertiaUnits=kg*m^2  ProductsOfInertia=[0 0 0]  ProductsOfInertiaUnits=kg*m^2  BasedOnType=Density  Density=1000  DensityUnits=kg/m^3  DoExposeReferenceFrame=off  SerializedFrames=<Frames><Frame><Id>Frame1</Id><Value><Name>F1</Name><Origin><Source>ReferenceFrame</Source><FeatureName></FeatureName></Origin><PrimaryAxis><DefinedDirection>+Z</DefinedDirection><Source>ReferenceFrame</Source><SourceDirection>+X</SourceDirection><FeatureName></FeatureName></PrimaryAxis><SecondaryAxis><DefinedDirection>+X</DefinedDirection><Source>ReferenceFrame</Source><SourceDirection>-Z</SourceDirection><FeatureName></FeatureName></SecondaryAxis></Value></Frame></Frames>  GraphicType=FromGeometry  MarkerShape=Sphere  MarkerSize=10  GraphicVisPropType=SimpleVisualProperties  GraphicDiffuseColor=[0.5 0.5 0.5]  GraphicSpecularColor=[0.5 0.5 0.5 1.0]  GraphicAmbientColor=[0.15 0.15 0.15 1.0]  GraphicEmissiveColor=[0.0 0.0 0.0 1.0]  GraphicShininess=75  GraphicOpacity=1.0
  "髋关节stl " : PMIOPort  Side=Left
  "大腿stl " : PMIOPort  Port=2  Side=Left
  "小腿stl " : PMIOPort  Port=3  Side=Left
  connections:
  "小腿stl "/RConn1 -- 小腿/LConn1
  "髋关节stl "/RConn1 -- 髋关节/LConn1
  "大腿stl "/RConn1 -- 左大腿/LConn1

== matlab function four_feet_simple_cdh/触地信号更新&状态机更新/触地信号更新&状态机更新 ==
  data: u1 output; u2 output; u3 output; u4 output; x1 input; y output; x2 input; x3 input; x4 input; S input; y2 output; uu input
function [u1,u2,u3,u4,y,y2] = fcn(x1,x2,x3,x4,S,uu)


force_threshold = 5;

if(x1>force_threshold)
    u1=1;
else
    u1=0;
end

if(x2>force_threshold)
    u2=1;
else
    u2=0;
end

if(x3>force_threshold)
    u3=1;
else
    u3=0;
end

if(x4>force_threshold)
    u4=1;
else
    u4=0;
end
%S=0,1,3抬腿，2,4支撑
%S=1,2,4抬腿，1,3支撑

y=S;
y2=uu;

%四足腾空相
if(u1==0  && u2==0  && u3==0  && u4==0 )
    y=-1;
    y2=uu+1;
end
%初始化并且全部触地
if(S==-1 && u1==1  && u2==1  && u3==1  && u4==1 )
    y=0;
    y2=uu+1;
end
%抬腿A组并且全部A组离地
if(S==0 && u2==1  && u4==1  && u1==0  && u3==0 )
    y=2;
end
%A组全部着地
if(S==2 && u1==1  && u2==1  && u3==1  && u4==1 )
    y=1;
     y2=uu+1;
end
%抬腿B组并且全部B组离地
if(S==1 && u1==1  && u3==1  && u2==0  && u4==0 )
    y=3;
end
%B组全部着地
if(S==3 && u1==1  && u2==1  && u3==1  && u4==1 )
    y=0;
    y2=uu+1;
end



end
